simulink model "lab1"  (R2023b)
settings: Solver=VariableStepAuto  StartTime=0.0  StopTime=10.0  FixedStep=0.1  MaxStep=10  RelTol=1e-3
model workspace (MAT data in the model file):
  Var = 0
undefined symbols (not defined in the file): cpw, Cvo1, Cvo2, delta_qt1, delta_qt2, delta_Twew_SP, delta_Tzew, deltafmg1, deltafmg2, fmg1_0, fmg2_0, fmw_0, Kco, ki2, kp2, qt1_0, qt2_0, t_fmg1, t_fmg2, T_gp0, t_op_tr, T_oz0, t_qt1, t_qt2, t_Twz, t_Tzew, t_wew_SP, T_wew_SP_0, T_wp0, T_wz, T_zew0
settings Model: Creator=tomasz  LastModifiedBy=tomasz

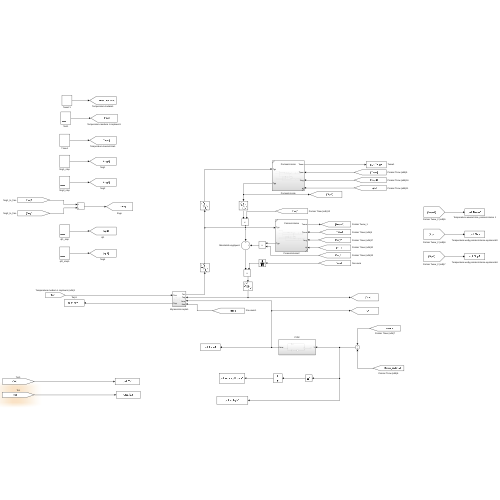
[thumbnail: Simulink's stored preview of the top-level diagram]
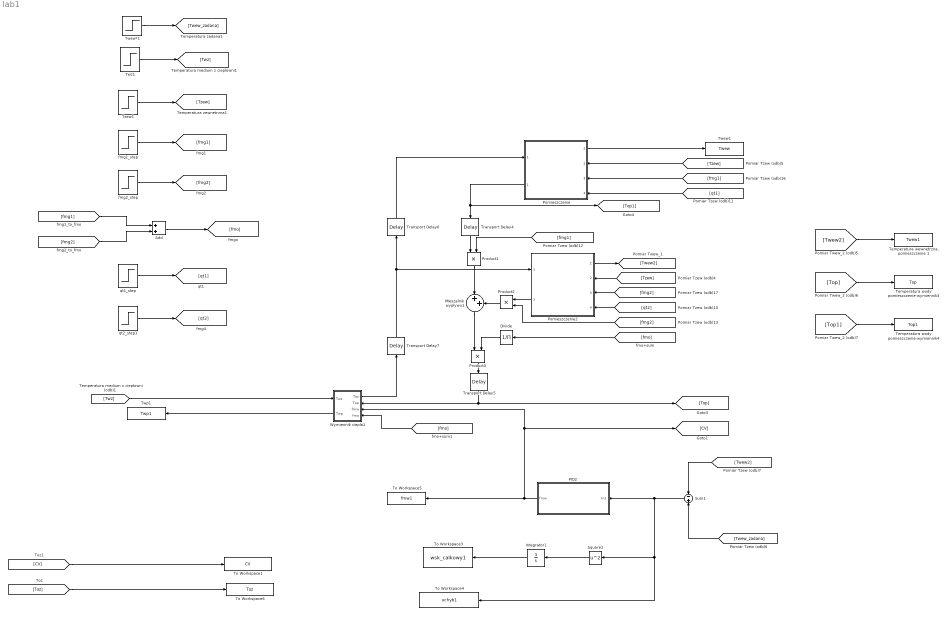
== system lab1 ==
  Add : Sum
  Divide : Product  Inputs=/
  Integrator1 : Integrator
  MIeszalnik wypływu1 : Sum  Inputs=|++
  PID2 : Subsystem
  Pomieszczenie : Subsystem  ReferencedSubsystem=Pomieszczenie
      settings: PortSchema="{\"entries\":[{\"content\":{\"sides\":[{\"content\":{\"connectorIds\":[\"In1\",\"Out1\"]},\"type\":\"ConnectorPlacement.EquallySpacedRectSide\",\"uuid\":\"8531bf00-72e2-4413-af12-728660d5b7ed\"},{\"content\":{\"connectorIds\":[\"Out2\",\"In2\",\"In3\",\"In4\"],\"side\":\"RIGHT\"},\"type\":\"ConnectorPlacement.EquallySpacedRectSide\",\"uuid\":\"61dc3c29-eecf-49ab-a3f8-5b1de1949346\"},{\"content\":{\"side\":\"TOP\"},\"type\":\"ConnectorPlacement.EquallySpacedRectSide\",\"uuid\":\"a446f5ea-277a-4598-bae9-2c6de6a131a4\"}]},\"type\":\"ConnectorPlacement.EquallySpacedConnector\",\"uuid\":\"c2b24185-542a-4b15-89a0-a367decd74d0\"}],\"packageUris\":[\"http://schema.mathworks.com/mf0/Connector/R2020b\"],\"version\":\"1.0\"}"
  Pomieszczenie2 : Subsystem  ReferencedSubsystem=Pomieszczenie
      settings: PortSchema="{\"entries\":[{\"content\":{\"sides\":[{\"content\":{\"connectorIds\":[\"In1\",\"Out1\"]},\"type\":\"ConnectorPlacement.EquallySpacedRectSide\",\"uuid\":\"8531bf00-72e2-4413-af12-728660d5b7ed\"},{\"content\":{\"connectorIds\":[\"Out2\",\"In2\",\"In3\",\"In4\"],\"side\":\"RIGHT\"},\"type\":\"ConnectorPlacement.EquallySpacedRectSide\",\"uuid\":\"61dc3c29-eecf-49ab-a3f8-5b1de1949346\"},{\"content\":{\"side\":\"TOP\"},\"type\":\"ConnectorPlacement.EquallySpacedRectSide\",\"uuid\":\"a446f5ea-277a-4598-bae9-2c6de6a131a4\"}]},\"type\":\"ConnectorPlacement.EquallySpacedConnector\",\"uuid\":\"c2b24185-542a-4b15-89a0-a367decd74d0\"}],\"packageUris\":[\"http://schema.mathworks.com/mf0/Connector/R2020b\"],\"version\":\"1.0\"}"
  Product1 : Product
  Product2 : Product
  Product3 : Product
  Square1 : Math  Operator=square
  Sum1 : Sum  Inputs=-+
  "Temperatura wewnetrzna, pomieszczenie 1" : ToWorkspace  VariableName=Twew1  SampleTime=-1
      settings: Save2DSignal=2-D array (concatenate along first dimension)
  Temperatura wody pomieszczenie-wymiennik3 : ToWorkspace  VariableName=Top  SampleTime=-1
      settings: Save2DSignal=2-D array (concatenate along first dimension)
  Temperatura wody pomieszczenie-wymiennik4 : ToWorkspace  VariableName=Top1  SaveFormat=Timeseries  SampleTime=-1
  To Workspace1 : ToWorkspace  VariableName=CV  SampleTime=-1
      settings: Save2DSignal=2-D array (concatenate along first dimension)
  To Workspace3 : ToWorkspace  VariableName=wsk_calkowy1  SampleTime=-1
  To Workspace4 : ToWorkspace  VariableName=uchyb1  SampleTime=-1
  To Workspace5 : ToWorkspace  VariableName=fmw1  SampleTime=-1
  To Workspace6 : ToWorkspace  VariableName=Toz  SampleTime=-1
  Transport Delay4 : TransportDelay  DelayTime=t_op_tr  InitialOutput=T_gp0
  Transport Delay5 : TransportDelay  DelayTime=t_op_tr  InitialOutput=T_gp0
  Transport Delay6 : TransportDelay  DelayTime=t_op_tr  InitialOutput=T_oz0
  Transport Delay7 : TransportDelay  DelayTime=t_op_tr  InitialOutput=T_oz0
  Twew*1 : Step  Time=t_wew_SP  Before=T_wew_SP_0  After=T_wew_SP_0 + delta_Twew_SP  SampleTime=0
  Twew1 : ToWorkspace  VariableName=Twew  SampleTime=-1
      settings: Save2DSignal=2-D array (concatenate along first dimension)
  Twp1 : ToWorkspace  VariableName=Twp1  SampleTime=-1
      settings: Save2DSignal=2-D array (concatenate along first dimension)
  Twz1 : Step  Time=t_Twz  Before=T_wz  After=T_wz  SampleTime=0
  Tzew1 : Step  Time=t_Tzew  Before=T_zew0  After=T_zew0 + delta_Tzew  SampleTime=0
  Wymiennik ciepla1 : Subsystem
      settings: PortSchema="{\"entries\":[{\"content\":{\"sides\":[{\"content\":{\"connectorIds\":[\"In1\",\"Out2\"]},\"type\":\"ConnectorPlacement.EquallySpacedRectSide\",\"uuid\":\"d2a1b48e-0b7a-4274-8a7b-b9fce30bfded\"},{\"content\":{\"connectorIds\":[\"Out1\",\"In2\",\"In3\",\"In4\"],\"side\":\"RIGHT\"},\"type\":\"ConnectorPlacement.EquallySpacedRectSide\",\"uuid\":\"703c2424-3a4a-4f57-8096-11f8c1d27324\"},{\"content\":{\"side\":\"TOP\"},\"type\":\"ConnectorPlacement.EquallySpacedRectSide\",\"uuid\":\"db7a7872-15b5-4367-ab72-78f604c615eb\"},{\"content\":{\"side\":\"BOTTOM\"},\"type\":\"ConnectorPlacement.EquallySpacedRectSide\",\"uuid\":\"9424703a-0ac4-48eb-878e-9dc2ecf23458\"}]},\"type\":\"ConnectorPlacement.EquallySpacedConnector\",\"uuid\":\"032bd106-566a-41c1-86c2-0fd4a1bc5877\"}],\"packageUris\":[\"http://schema.mathworks.com/mf0/Connector/R2020b\"],\"version\":\"1.0\"}"
  fmg1_step : Step  Time=t_fmg1  Before=fmg1_0  After=fmg1_0 + deltafmg1  SampleTime=0
  fmg2_step : Step  Time=t_fmg2  Before=fmg2_0  After=fmg2_0 + deltafmg2  SampleTime=0
  qt1_step : Step  Time=t_qt1  Before=qt1_0  After=qt1_0 + delta_qt1  SampleTime=0
  qt2_step1 : Step  Time=t_qt2  Before=qt2_0  After=qt2_0 + delta_qt2  SampleTime=0
  wires:
  Transport Delay5/1 -> [Top], Wymiennik ciepla1/2(Top)
  [Top] -> Temperatura wody pomieszczenie-wymiennik3/1
  [Tzew] -> Pomieszczenie/2
  [fmg2] -> Add/2
  [Tzew] -> Pomieszczenie2/2
  [Twew2] -> "Temperatura wewnetrzna, pomieszczenie 1"/1
  [Twew2] -> Sum1/1
  Product2/1 -> MIeszalnik wypływu1/2
  [qt1] -> Pomieszczenie/4
  [qt2] -> Pomieszczenie2/4
  Square1/1 -> Integrator1/1
  [fmg1] -> Product1/2
  [Toz] -> To Workspace6/1
  Wymiennik ciepla1/2(Twp) -> Twp1/1
  MIeszalnik wypływu1/1 -> Product3/1
  Pomieszczenie2/1 -> Product2/1
  [fmg1] -> Pomieszczenie/3
  qt2_step1/1 -> [qt2]
  qt1_step/1 -> [qt1]
  [Twew_zadana] -> Sum1/2
  Divide/1 -> Product3/2
  Product1/1 -> MIeszalnik wypływu1/1
  Tzew1/1 -> [Tzew]
  Transport Delay6/1 -> Pomieszczenie/1
  [fmo] -> Wymiennik ciepla1/4(fmo)
  Transport Delay7/1 -> Transport Delay6/1, Pomieszczenie2/1
  fmg2_step/1 -> [fmg2]
  [fmo] -> Divide/1
  Transport Delay4/1 -> Product1/1
  Pomieszczenie/1 -> Transport Delay4/1, [Top1]
  fmg1_step/1 -> [fmg1]
  PID2/1(fmw) -> [CV], Wymiennik ciepla1/3(fmw), To Workspace5/1
  [fmg2] -> Pomieszczenie2/3
  Twew*1/1 -> [Twew_zadana]
  [fmg2] -> Product2/2
  Pomieszczenie/2 -> Twew1/1
  Pomieszczenie2/2 -> [Twew2]
  Product3/1 -> Transport Delay5/1
  [Top1] -> Temperatura wody pomieszczenie-wymiennik4/1
  Sum1/1 -> PID2/1(In1), Square1/1, To Workspace4/1
  Add/1 -> [fmo]
  [fmg1] -> Add/1
  Wymiennik ciepla1/1(Toz) -> Transport Delay7/1
  Integrator1/1 -> To Workspace3/1
  [Twz] -> Wymiennik ciepla1/1(Twz)
  Twz1/1 -> [Twz]
  [CV] -> To Workspace1/1

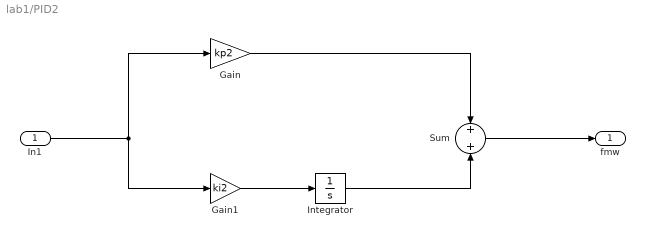
== system lab1/PID2 ==
  In1 : Inport
  Gain : Gain  Gain=kp2
  Gain1 : Gain  Gain=ki2
  Integrator : Integrator  InitialCondition=fmw_0
  Sum : Sum
  fmw : Outport
  wires:
  Gain1/1 -> Integrator/1
  Gain/1 -> Sum/1
  In1/1 -> Gain1/1, Gain/1
  Integrator/1 -> Sum/2
  Sum/1 -> fmw/1

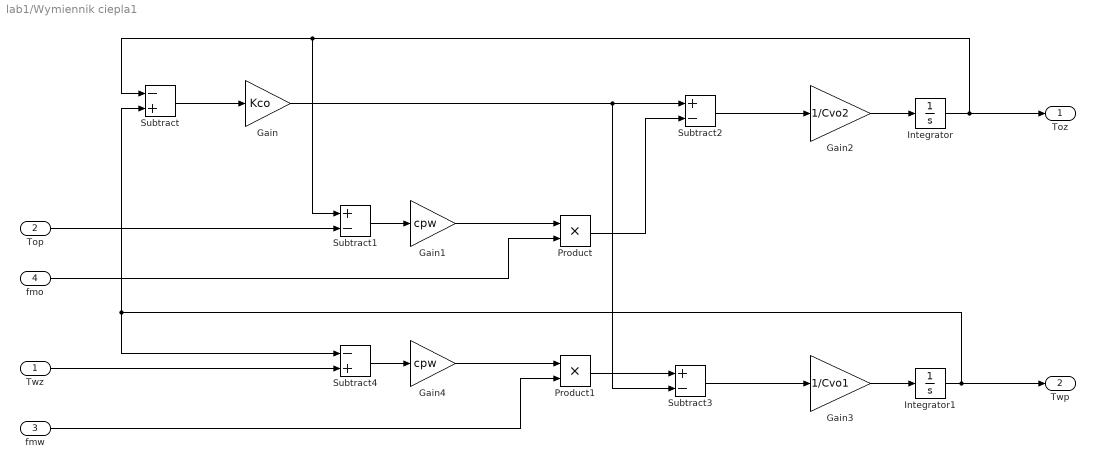
== system lab1/Wymiennik ciepla1 ==
  Twz : Inport
  Top : Inport  Port=2
  fmw : Inport  Port=3
  fmo : Inport  Port=4
  Gain : Gain  Gain=Kco
  Gain1 : Gain  Gain=cpw
  Gain2 : Gain  Gain=1/Cvo2
  Gain3 : Gain  Gain=1/Cvo1
  Gain4 : Gain  Gain=cpw
  Integrator : Integrator  InitialCondition=T_oz0
  Integrator1 : Integrator  InitialCondition=T_wp0
  Product : Product
  Product1 : Product
  Subtract : Sum  Inputs=-+
  Subtract1 : Sum  Inputs=+-
  Subtract2 : Sum  Inputs=+-
  Subtract3 : Sum  Inputs=+-
  Subtract4 : Sum  Inputs=-+
  Toz : Outport
  Twp : Outport  Port=2
  wires:
  Gain4/1 -> Product1/1
  Gain3/1 -> Integrator1/1
  fmw/1 -> Product1/2
  Product/1 -> Subtract2/2
  Product1/1 -> Subtract3/1
  Integrator1/1 -> Twp/1, Subtract/2, Subtract4/1
  Gain2/1 -> Integrator/1
  Subtract4/1 -> Gain4/1
  Gain/1 -> Subtract3/2, Subtract2/1
  Top/1 -> Subtract1/2
  Subtract3/1 -> Gain3/1
  Subtract/1 -> Gain/1
  Gain1/1 -> Product/1
  Twz/1 -> Subtract4/2
  Subtract2/1 -> Gain2/1
  Subtract1/1 -> Gain1/1
  fmo/1 -> Product/2
  Integrator/1 -> Toz/1, Subtract1/1, Subtract/1
